simulink model "traffic_signal"  (R2024b)
settings: Solver=FixedStepDiscrete  StartTime=0.0  StopTime=300  FixedStep=1  RelTol=1e-3

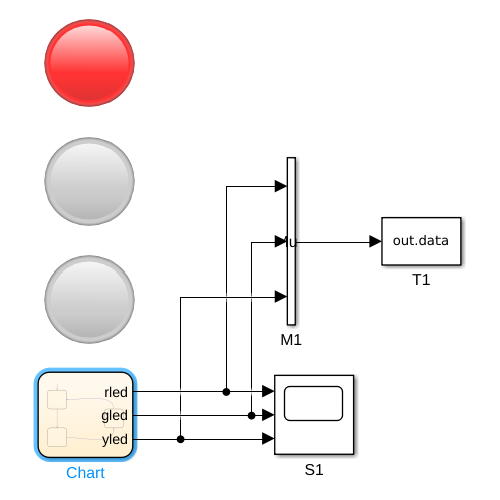
[thumbnail: Simulink's stored preview of the top-level diagram]
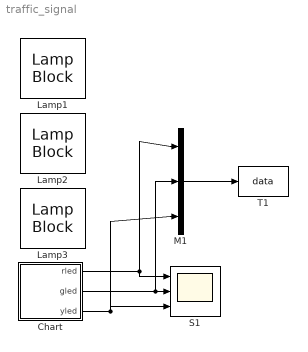
== system traffic_signal ==
  Chart : Stateflow chart  TreatAsAtomicUnit=on
  Lamp1 : LampBlock  LabelPosition=Hide
  Lamp2 : LampBlock  LabelPosition=Hide
  Lamp3 : LampBlock  LabelPosition=Hide
  M1 : Mux  Inputs=3
  S1 : Scope  NumInputPorts=3
  T1 : ToWorkspace  VariableName=data  SaveFormat=Structure With Time
  wires:
  M1/1 -> T1/1
  Chart/3(yled) -> M1/3, S1/3
  Chart/2(gled) -> M1/2, S1/2
  Chart/1(rled) -> M1/1, S1/1

== stateflow chart traffic_signal/Chart ==
  state Red
    during:
    rled = 1;
    exit:
    rled = 0;
  state Yellow
    during:
    yled = 1;
    exit:
    yled = 0;
  state Green
    during:
    gled = 1;
    exit:
    gled = 0;
  (default) -> Red
  Yellow -> Red : after(5,sec)
  Red -> Green : after(30,sec)
  Green -> Yellow : after(25,sec)
  data: rled output single; gled output single; yled output single
